simulink subsystem "Vehicle_Model"  (R2022b)
settings: Solver=VariableStepAuto  StartTime=0.0  StopTime=10.0  RelTol=1e-3
undefined symbols (not defined in the file): chassis, dZ, F0z, IMU_accel, IMU_gyro, IMU_mag, phi, powertrain, psi, sim, sus, suspension, theta, trn, veh, VEH, whl, X, Xdot, Y, Ydot, Z, Zdot
libraries: fl_lib x53, nesl_utility x15, vehdynlibtire x10, vehdynlibsuspension x8, EngineCoolingComponents_lib x5, autolibutils x5, sharedtransform x5, shared6dof x2, sensorgpslib x1, mspsensorlib x1, dspstat3 x1, SimscapeFluids_lib x1
(part 8 of 8)

== system Vehicle_Model/Wheels and Tires/VDBS/Tires/MF Tires Vector ==
  DriveTorque : Inport
  Brake Pedal : Inport  Port=2
  r : Inport  Port=3
  Vx : Inport  Port=4
  Vy : Inport  Port=5
  Camber : Inport  Port=6
  Press : Inport  Port=7  Unit=Pa
  lambda : Inport  Port=8  Unit=1
  Gnd : Inport  Port=9
  FzSusp : Inport  Port=10
  Combined Slip Wheel 2DOF : vehdynlibtire/Combined Slip Wheel 2DOF  plySteer=on  turnslip=on  tireType=External file  BrakeType=Disc  mu_static=powertrain.brake.mu_static  mu_kinetic=powertrain.brake.mu_kinetic  disk_abore=powertrain.brake.disk_abore  Rm=powertrain.brake.Rm  num_pads=powertrain.brake.num_pads  drum_abore=0.0508  drum_a=0.123  drum_c=0.212  drum_r=0.15  drum_theta1=0  drum_theta2=126  brake_p_bpt=[1 11.4736842105263 21.9473684210526 32.4210526315789 42.8947368421053 53.3684210526316 63.8421052631579 74.3157894736842 84.7894736842105 95.2631578947368 105.736842105263 116.210526315789 126.684210526316 137.157894736842 147.631578947368 158.105263157895 168.578947368421 179.052631578947 189.526315789474 200]  brake_n_bpt=[0 52.6315789473684 105.263157894737 157.894736842105 210.526315789474 263.157894736842 315.789473684211 368.421052631579 421.052631578947 473.684210526316 526.315789473684 578.947368421053 631.578947368421 684.210526315789 736.842105263158 789.473684210526 842.105263157895 894.736842105263 947.368421052632 1000]  f_brake_t=[43.4900602404453 42.5056030554862 41.5350898940194 40.5780454442085 39.6340111501808 38.7025443887544 37.7832176914519 36.8756180088306 35.9793460143796 35.0940154454303 34.2192524787115 33.3546951383474 32.4999927342521 31.6548053290159 30.8188032315107 29.991666515561 29.1730845621415 28.362755623661 27.5603864089927 26.765691687993;498.991217495636 487.695866636631 476.560505099801 465.579679307235 454.748127933653 444.060772460445 433.51270824929 423.099196101319 412.81565427025 402.657650900201 392.620896861006 382.701238955775 372.894653477208 363.197240090814 353.605216024701 344.114910546964 334.722759712992 325.425301366216 316.219170376863 307.10109410434;954.492374750826 932.886130217776 911.585920305583 890.581313170261 869.862244717126 849.419000532136 829.242198807128 809.322774193808 789.651962526121 770.221286354971 751.0225412433 732.047782773203 713.289314220164 694.739674852612 676.391628817892 658.238154578366 640.272434863842 622.48784710877 604.877954344734 587.436496520688;1409.99353200602 1378.07639379892 1346.61133551136 1315.58294703329 1284.9763615006 1254.77722860383 1224.97168936497 1195.5463522863 1166.48827078199 1137.78492180974 1109.42418562559 1081.39432659063 1053.68397496312 1026.28210961441 999.178041611083 972.361398609768 945.822110014692 919.550392851325 893.536738312604 867.771898937035;1865.49468926121 1823.26665738007 1781.63675071715 1740.58458089631 1700.09047828407 1660.13545667552 1620.7011799228 1581.76993037878 1543.32457903786 1505.34855726451 1467.82583000789 1430.74087040806 1394.07863570608 1357.82454437621 1321.96445440427 1286.48464264117 1251.37178516554 1216.61293859388 1182.19552228048 1148.10730135338;2320.9958465164 2268.45692096121 2216.66216592293 2165.58621475934 2115.20459506754 2065.49368474721 2016.43067048064 1967.99350847127 1920.16088729373 1872.91219271928 1826.22747439018 1780.08741422549 1734.47329644903 1689.36697913801 1644.75086719747 1600.60788667257 1556.92146031639 1513.67548433643 1470.85430624835 1428.44270376973;2776.49700377159 2713.64718454235 2651.68758112871 2590.58784862237 2530.31871185102 2470.8519128189 2412.16016103848 2354.21708656376 2296.9971955496 2240.47582817405 2184.62911877248 2129.43395804292 2074.86795719199 2020.9094138998 1967.53727999066 1914.73113070398 1862.47113546724 1810.73803007899 1759.51309021622 1708.77810618608;3231.99816102678 3158.8374481235 3086.71299633449 3015.58948248539 2945.43282863449 2876.21014089059 2807.88965159632 2740.44066465625 2673.83350380547 2608.03946362882 2543.03076315477 2478.78050186034 2415.26261793494 2352.4518486616 2290.32369278385 2228.85437473538 2168.02081061809 2107.80057582154 2048.17187418409 1989.11350860242;3687.49931828197 3604.02771170464 3521.73841154027 3440.59111634842 3360.54694541796 3281.56836896228 3203.61914215416 3126.66424274874 3050.66981206134 2975.60309908359 2901.43240753707 2828.12704567777 2755.6572786779 2683.9942834234 2613.11010557704 2542.97761876678 2473.57048576894 2404.8631215641 2336.83065815196 2269.44891101877;4143.00047553716 4049.21797528579 3956.76382674606 3865.59275021144 3775.66106220143 3686.92659703397 3599.34863271199 3512.88782084123 3427.50612031721 3343.16673453836 3259.83405191936 3177.4735894952 3096.05193942085 3015.5367181852 2935.89651837023 2857.10086279818 2779.12016091979 2701.92566730665 2625.48944211983 2549.78431343512;4598.50163279235 4494.40823886693 4391.78924195184 4290.59438407447 4190.77517898491 4092.28482510566 3995.07812326983 3899.11139893372 3804.34242857308 3710.73036999313 3618.23569630166 3526.82013331263 3436.44660016381 3347.079152947 3258.68293116342 3171.22410682959 3084.66983607064 2998.98821304921 2914.1482260877 2830.11971585147;5054.00279004754 4939.59850244808 4826.81465715762 4715.59601793749 4605.88929576838 4497.64305317735 4390.80761382767 4285.3349770262 4181.17873682896 4078.2940054479 3976.63734068395 3876.16667713006 3776.84126090677 3678.62158770879 3581.46934395661 3485.34735086099 ...(+2764 chars)]  tireParamSet=C:\Users\Inver\Documents\GitHub\SimscapeModel\Vehicle Parameters\PROCESSED_DATA\Round_6_Hoosier_LCO_18x6_10_on_6in_12psi_PAC02_UM4.tir  PRESMAX=1000000  PRESMIN=10000  FZMAX=1121  FZMIN=10  VXLOW=1  KPUMAX=0.25  KPUMIN=-0.25  ALPMAX=0.261799  ALPMIN=-0.261799  CAMMAX=0.069813  CAMMIN=-0.069813  LONGVL=11.176  FxRelFreqLwrLim=200*pi  FyRelFreqLwrLim=50*pi  MyRelFreqLwrLim=100*pi  omegao=sim.IC.omega_IC  br=suspension.tire.br  UNLOADED_RADIUS=0.2286  NOMPRES=sim.strange_parameters.NOMPRES  FNOMIN=601  WIDTH=0.1524  RIM_RADIUS=0.127  MASS=mean(chassis.mass.m_unsprung)  IYY=suspension.tire.IYY  GRAVITY=-sim.constant.g  zo=sim.IC.z_tire_IC  zdoto=sim.IC.zdot_tires_IC  BREFF=2.49297  DREFF=0.321682  FREFF=0.251668  Q_RE0=1.00866439868088  Q_V1=0.000760413786224011  Q_V2=0.0463384792019201  Q_FZ1=0  Q_FZ2=15.6870832810226  Q_FZ3=0  Q_FCX=0.138643970247602  Q_FCY=0.10843499565426  Q_FCY2=-0.465763352339538  PFZ1=0.69958166705601  VERTICAL_STIFFNESS=112400  VERTICAL_DAMPING=118.254  BOTTOM_OFFST=0.00990653336182505  BOTTOM_STIFF=1999075.87051971  LONGITUDINAL_STIFFNESS=388714.175879854  LATERAL_STIFFNESS=157087.404633332  PCFX1=0.18539229191199  PCFX2=0  PCFX3=0  PCFY1=0.163183345037677  PCFY2=0  PCFY3=0.249094918231954  Q_RA1=0.675942571700787  Q_RA2=0.73800463546164  Q_RB1=1.04487486456705  Q_RB2=-1.191763806629  PCX1=0.966202  PDX1=2.80407  PDX2=-0.357084  PDX3=6.84244  PEX1=-6.80827e-05  PEX2=-1.03475  PEX3=-0.53468  PEX4=-1  PKX1=54.4164  PKX2=-22.3491  PKX3=0.0455377  PHX1=0.00128776  PHX2=0.00137717  PVX1=-0.0646749  PVX2=-0.100465  PPX1=0  PPX2=0  PPX3=0  PPX4=0  RBX1=100  RBX2=44.8344  RBX3=0  RCX1=0.856322  REX1=0.518432  REX2=0.240784  RHX1=-0.0150667  QSX1=-0.0194497  QSX2=-1.24676  QSX3=0.000838911  QSX4=0.807548  QSX5=-0.37375  QSX6=1.16556  QSX7=-5.15598  QSX8=-0.492061  QSX9=-0.177936  QSX10=1  QSX11=0.888738  QSX12=0  QSX13=0  QSX14=0  PPMX1=0  PCY1=0.752535  PDY1=-3.27392  PDY2=0.218557  PDY3=6.02342  PEY1=0  PEY2=0.252909  PEY3=-0.706443  PEY4=0.9  PEY5=0  PKY1=-48.6492  PKY2=1.68896  PKY3=1.62566  PKY4=1.98176755955416  PKY5=0  PKY6=-0.884005199550313  PKY7=-0.237259727611847  PHY1=0.0017727  PHY2=-0.00215785  PVY1=0.0212074  PVY2=-0.0480939  PVY3=0.200755  PVY4=-1.48156  PPY1=0  PPY2=0  PPY3=0  PPY4=0  PPY5=0  RBY1=12.042  RBY2=10.4  RBY3=-0.0251847  RBY4=0  RCY1=1.05268  REY1=-0.0970159  REY2=-0.211702  RHY1=0.00468209  RHY2=0.0130759  RVY1=0.00281892  RVY2=-0.0024726  RVY3=-0.0308756  RVY4=-50  RVY5=-3  RVY6=22  QSY1=0  QSY2=0  QSY3=0  QSY4=0  QSY5=0  QSY6=0  QSY7=0  QSY8=0  QBZ1=7.76297  QBZ2=1.09215  QBZ3=-0.949071  QBZ4=9.45639  QBZ5=-9.95728  QBZ6=0  QBZ9=0  QBZ10=2.46233  QCZ1=1.1619  QDZ1=0.130674  QDZ2=-0.0191515  QDZ3=-2.11221  QDZ4=4.36886  QDZ6=0.00252395  QDZ7=0.0164922  QDZ8=-1.57877  QDZ9=0.435267  QDZ10=0  QDZ11=0  QEZ1=-2.11897  QEZ2=0.850576  QEZ3=0.223032  QEZ4=0.657831  QEZ5=-7.10343  QHZ1=0.00740081  QHZ2=-0.00996544  QHZ3=0.0623105  QHZ4=-0.331019  PPZ1=-0.443927982388615  PPZ2=0  SSZ1=-0.0881802  SSZ2=-0.0389434  SSZ3=1.55783  SSZ4=-0.570516  PDXP1=0.396718274678791  PDXP2=0  PDXP3=0  PKYP1=1.00587060633573  PDYP1=0.40483048923438  PDYP2=0  PDYP3=0  PDYP4=0  PHYP1=0.992731942067188  PHYP2=0.150352945499914  PHYP3=0  PHYP4=-3.98988682633674  PECP1=0.502379254513503  PECP2=0  QDTP1=10.0178654287947  QCRP1=0.200627747200702  QCRP2=0.0995735881599772  QBRP1=0.0997107127960717  QDRP1=1.01432910167423  QDRP2=0  aMode=2
  Terminator{7..13} (7 alike) : Terminator
  Wheels : Outport  VectorParamsAs1DForOutWhenUnconnected=off
  wires:
  lambda/1 -> Combined Slip Wheel 2DOF/10
  Combined Slip Wheel 2DOF/1 -> Wheels/1
  DriveTorque/1 -> Combined Slip Wheel 2DOF/2
  Vx/1 -> Combined Slip Wheel 2DOF/3
  Camber/1 -> Combined Slip Wheel 2DOF/5
  r/1 -> Combined Slip Wheel 2DOF/6
  Press/1 -> Combined Slip Wheel 2DOF/7
  Gnd/1 -> Combined Slip Wheel 2DOF/8
  FzSusp/1 -> Combined Slip Wheel 2DOF/9
  Combined Slip Wheel 2DOF/2 -> Terminator7/1
  Combined Slip Wheel 2DOF/3 -> Terminator8/1
  Combined Slip Wheel 2DOF/4 -> Terminator9/1
  Combined Slip Wheel 2DOF/5 -> Terminator10/1
  Combined Slip Wheel 2DOF/6 -> Terminator11/1
  Combined Slip Wheel 2DOF/7 -> Terminator12/1
  Combined Slip Wheel 2DOF/8 -> Terminator13/1
  Vy/1 -> Combined Slip Wheel 2DOF/4
  Brake Pedal/1 -> Combined Slip Wheel 2DOF/1

== system Vehicle_Model/Wheels and Tires/VDBS/Veh2Tire/Wheel Angles ==
  steer : Inport
  camber : Inport  Port=2
  Constant3 : Constant  Value=ones(1,4).*0
  Reshape : Reshape  OutputDimensionality=Row vector (2-D)
  Reshape1 : Reshape  OutputDimensionality=Row vector (2-D)
  Reshape2 : Reshape  OutputDimensionality=Row vector (2-D)
  Vector Concatenate3 : Concatenate  NumInputs=3  Mode=Multidimensional array
  Vehicle : Outport  VectorParamsAs1DForOutWhenUnconnected=off
  wires:
  Constant3/1 -> Reshape2/1
  Vector Concatenate3/1 -> Vehicle/1
  Reshape/1 -> Vector Concatenate3/3
  Reshape1/1 -> Vector Concatenate3/1
  camber/1 -> Reshape1/1
  Reshape2/1 -> Vector Concatenate3/2
  steer/1 -> Reshape/1

== system Vehicle_Model/Wheels and Tires/VDBS/Veh2Tire/Wheel to Body Transform ==
  VelVeh : Inport  Partition=on  PartitionDimension=2  PartitionWidth=1  PartitionOffset=0
  WheelAngles : Inport  Port=2  Partition=on  PartitionDimension=2  PartitionWidth=1  PartitionOffset=0
  Constant : Constant  Value=[pi;0;0]
  Demux1 : Demux  Outputs=3
  Divide1 : Product  Inputs=**  Multiplication=Matrix(*)
  Divide2 : Product  Inputs=**  Multiplication=Matrix(*)
  For Each : ForEach  DisableCoverage=on
  Rotation Angles to Direction Cosine Matrix : sharedtransform/Rotation Angles to Direction Cosine Matrix  rotationOrder=ZYX  aMode=2
  Rotation Angles to Direction Cosine Matrix1 : sharedtransform/Rotation Angles to Direction Cosine Matrix  rotationOrder=ZYX  aMode=2
  Selector : Selector  InputPortWidth=3  IndexOptions=Index vector (dialog)  Indices=[3 2 1]  OutputSizes=1
  Selector1 : Selector  InputPortWidth=3  IndexOptions=Index vector (dialog)  Indices=[3 2 1]  OutputSizes=1
  xdotWheel : Outport  ConcatenationDimension=1  VectorParamsAs1DForOutWhenUnconnected=off
  ydotWheel : Outport  Port=2  ConcatenationDimension=1  VectorParamsAs1DForOutWhenUnconnected=off
  zdotWheel : Outport  Port=3  ConcatenationDimension=1  VectorParamsAs1DForOutWhenUnconnected=off
  wires:
  Divide2/1 -> Demux1/1
  Demux1/1 -> xdotWheel/1
  Demux1/2 -> ydotWheel/1
  Demux1/3 -> zdotWheel/1
  Rotation Angles to Direction Cosine Matrix/1 -> Divide1/1
  VelVeh/1 -> Divide1/2
  WheelAngles/1 -> Selector/1
  Selector/1 -> Rotation Angles to Direction Cosine Matrix/1
  Selector1/1 -> Rotation Angles to Direction Cosine Matrix1/1
  Rotation Angles to Direction Cosine Matrix1/1 -> Divide2/1
  Divide1/1 -> Divide2/2
  Constant/1 -> Selector1/1

== system Vehicle_Model/Wheels and Tires/VDBS/Tires/Fiala Tires/Fx ==
  In1 : Inport
  In2 : Inport  Port=2
  In3 : Inport  Port=3
  In4 : Inport  Port=4
  Bus Selector{,1..3} (4 alike) : BusSelector  OutputSignals=Fx
  Vector Concatenate : Concatenate  NumInputs=4
  Out1 : Outport  VectorParamsAs1DForOutWhenUnconnected=off
  wires:
  Bus Selector3/1 -> Vector Concatenate/4  "<Fx>"
  Bus Selector2/1 -> Vector Concatenate/3  "<Fx>"
  Bus Selector1/1 -> Vector Concatenate/2  "<Fx>"
  In4/1 -> Bus Selector3/1
  In3/1 -> Bus Selector2/1
  In2/1 -> Bus Selector1/1
  Bus Selector/1 -> Vector Concatenate/1  "<Fx>"
  In1/1 -> Bus Selector/1
  Vector Concatenate/1 -> Out1/1

== system Vehicle_Model/Wheels and Tires/VDBS/Tires/Fiala Tires/Fy ==
  In1 : Inport
  In2 : Inport  Port=2
  In3 : Inport  Port=3
  In4 : Inport  Port=4
  Bus Selector{,1..3} (4 alike) : BusSelector  OutputSignals=Fy
  Vector Concatenate : Concatenate  NumInputs=4
  Out1 : Outport  VectorParamsAs1DForOutWhenUnconnected=off
  wires:
  Vector Concatenate/1 -> Out1/1
  In1/1 -> Bus Selector/1
  Bus Selector/1 -> Vector Concatenate/1  "<Fy>"
  In2/1 -> Bus Selector1/1
  In3/1 -> Bus Selector2/1
  In4/1 -> Bus Selector3/1
  Bus Selector1/1 -> Vector Concatenate/2  "<Fy>"
  Bus Selector2/1 -> Vector Concatenate/3  "<Fy>"
  Bus Selector3/1 -> Vector Concatenate/4  "<Fy>"

== system Vehicle_Model/Wheels and Tires/VDBS/Tires/Fiala Tires/Fz ==
  In1 : Inport
  In2 : Inport  Port=2
  In3 : Inport  Port=3
  In4 : Inport  Port=4
  Bus Selector{,1..3} (4 alike) : BusSelector  OutputSignals=Fz
  Vector Concatenate : Concatenate  NumInputs=4
  Out1 : Outport  VectorParamsAs1DForOutWhenUnconnected=off
  wires:
  Vector Concatenate/1 -> Out1/1
  In1/1 -> Bus Selector/1
  Bus Selector/1 -> Vector Concatenate/1  "<Fz>"
  In2/1 -> Bus Selector1/1
  In3/1 -> Bus Selector2/1
  In4/1 -> Bus Selector3/1
  Bus Selector1/1 -> Vector Concatenate/2  "<Fz>"
  Bus Selector2/1 -> Vector Concatenate/3  "<Fz>"
  Bus Selector3/1 -> Vector Concatenate/4  "<Fz>"

== system Vehicle_Model/Wheels and Tires/VDBS/Tires/Fiala Tires/Mx ==
  In1 : Inport
  In2 : Inport  Port=2
  In3 : Inport  Port=3
  In4 : Inport  Port=4
  Bus Selector{,1..3} (4 alike) : BusSelector  OutputSignals=Mx
  Vector Concatenate : Concatenate  NumInputs=4
  Out1 : Outport  VectorParamsAs1DForOutWhenUnconnected=off
  wires:
  Vector Concatenate/1 -> Out1/1
  In1/1 -> Bus Selector/1
  Bus Selector/1 -> Vector Concatenate/1  "<Mx>"
  In2/1 -> Bus Selector1/1
  In3/1 -> Bus Selector2/1
  In4/1 -> Bus Selector3/1
  Bus Selector1/1 -> Vector Concatenate/2  "<Mx>"
  Bus Selector2/1 -> Vector Concatenate/3  "<Mx>"
  Bus Selector3/1 -> Vector Concatenate/4  "<Mx>"

== system Vehicle_Model/Wheels and Tires/VDBS/Tires/Fiala Tires/My ==
  In1 : Inport
  In2 : Inport  Port=2
  In3 : Inport  Port=3
  In4 : Inport  Port=4
  Bus Selector{,1..3} (4 alike) : BusSelector  OutputSignals=My
  Vector Concatenate : Concatenate  NumInputs=4
  Out1 : Outport  VectorParamsAs1DForOutWhenUnconnected=off
  wires:
  Bus Selector3/1 -> Vector Concatenate/4  "<My>"
  Bus Selector2/1 -> Vector Concatenate/3  "<My>"
  Bus Selector1/1 -> Vector Concatenate/2  "<My>"
  In4/1 -> Bus Selector3/1
  In3/1 -> Bus Selector2/1
  In2/1 -> Bus Selector1/1
  Bus Selector/1 -> Vector Concatenate/1  "<My>"
  In1/1 -> Bus Selector/1
  Vector Concatenate/1 -> Out1/1

== system Vehicle_Model/Wheels and Tires/VDBS/Tires/Fiala Tires/Mz ==
  In1 : Inport
  In2 : Inport  Port=2
  In3 : Inport  Port=3
  In4 : Inport  Port=4
  Bus Selector{,1..3} (4 alike) : BusSelector  OutputSignals=Mz
  Vector Concatenate : Concatenate  NumInputs=4
  Out1 : Outport  VectorParamsAs1DForOutWhenUnconnected=off
  wires:
  Bus Selector3/1 -> Vector Concatenate/4  "<Mz>"
  Bus Selector2/1 -> Vector Concatenate/3  "<Mz>"
  Bus Selector1/1 -> Vector Concatenate/2  "<Mz>"
  In4/1 -> Bus Selector3/1
  In3/1 -> Bus Selector2/1
  In2/1 -> Bus Selector1/1
  Bus Selector/1 -> Vector Concatenate/1  "<Mz>"
  In1/1 -> Bus Selector/1
  Vector Concatenate/1 -> Out1/1

== system Vehicle_Model/Wheels and Tires/VDBS/Tires/Fiala Tires/Re ==
  In1 : Inport
  In2 : Inport  Port=2
  In3 : Inport  Port=3
  In4 : Inport  Port=4
  Bus Selector{,1..3} (4 alike) : BusSelector  OutputSignals=Re
  Vector Concatenate : Concatenate  NumInputs=4
  Out1 : Outport  VectorParamsAs1DForOutWhenUnconnected=off
  wires:
  Vector Concatenate/1 -> Out1/1
  In1/1 -> Bus Selector/1
  Bus Selector/1 -> Vector Concatenate/1  "<Re>"
  In2/1 -> Bus Selector1/1
  In3/1 -> Bus Selector2/1
  In4/1 -> Bus Selector3/1
  Bus Selector1/1 -> Vector Concatenate/2  "<Re>"
  Bus Selector2/1 -> Vector Concatenate/3  "<Re>"
  Bus Selector3/1 -> Vector Concatenate/4  "<Re>"

== system Vehicle_Model/Wheels and Tires/VDBS/Tires/Fiala Tires/alpha ==
  In1 : Inport
  In2 : Inport  Port=2
  In3 : Inport  Port=3
  In4 : Inport  Port=4
  Bus Selector{,1..3} (4 alike) : BusSelector  OutputSignals=Alpha
  Vector Concatenate : Concatenate  NumInputs=4
  Out1 : Outport  VectorParamsAs1DForOutWhenUnconnected=off
  wires:
  Vector Concatenate/1 -> Out1/1
  In1/1 -> Bus Selector/1
  Bus Selector/1 -> Vector Concatenate/1  "<Alpha>"
  In2/1 -> Bus Selector1/1
  In3/1 -> Bus Selector2/1
  In4/1 -> Bus Selector3/1
  Bus Selector1/1 -> Vector Concatenate/2  "<Alpha>"
  Bus Selector2/1 -> Vector Concatenate/3  "<Alpha>"
  Bus Selector3/1 -> Vector Concatenate/4  "<Alpha>"

== system Vehicle_Model/Wheels and Tires/VDBS/Tires/Fiala Tires/kappa ==
  In1 : Inport
  In2 : Inport  Port=2
  In3 : Inport  Port=3
  In4 : Inport  Port=4
  Bus Selector{,1..3} (4 alike) : BusSelector  OutputSignals=Kappa
  Vector Concatenate : Concatenate  NumInputs=4
  Out1 : Outport  VectorParamsAs1DForOutWhenUnconnected=off
  wires:
  Bus Selector3/1 -> Vector Concatenate/4  "<Kappa>"
  Bus Selector2/1 -> Vector Concatenate/3  "<Kappa>"
  Bus Selector1/1 -> Vector Concatenate/2  "<Kappa>"
  In4/1 -> Bus Selector3/1
  In3/1 -> Bus Selector2/1
  In2/1 -> Bus Selector1/1
  Bus Selector/1 -> Vector Concatenate/1  "<Kappa>"
  In1/1 -> Bus Selector/1
  Vector Concatenate/1 -> Out1/1

== system Vehicle_Model/Wheels and Tires/VDBS/Tires/Fiala Tires/omega ==
  In1 : Inport
  In2 : Inport  Port=2
  In3 : Inport  Port=3
  In4 : Inport  Port=4
  Bus Selector{,1..3} (4 alike) : BusSelector  OutputSignals=Omega
  Vector Concatenate : Concatenate  NumInputs=4
  Out1 : Outport  VectorParamsAs1DForOutWhenUnconnected=off
  wires:
  In1/1 -> Bus Selector/1
  Bus Selector/1 -> Vector Concatenate/1  "<Omega>"
  In2/1 -> Bus Selector1/1
  In3/1 -> Bus Selector2/1
  In4/1 -> Bus Selector3/1
  Bus Selector1/1 -> Vector Concatenate/2  "<Omega>"
  Bus Selector2/1 -> Vector Concatenate/3  "<Omega>"
  Bus Selector3/1 -> Vector Concatenate/4  "<Omega>"
  Vector Concatenate/1 -> Out1/1

== system Vehicle_Model/Wheels and Tires/VDBS/Tires/Fiala Tires/z ==
  In1 : Inport
  In2 : Inport  Port=2
  In3 : Inport  Port=3
  In4 : Inport  Port=4
  Bus Selector{,1..3} (4 alike) : BusSelector  OutputSignals=z
  Vector Concatenate : Concatenate  NumInputs=4
  Out1 : Outport  VectorParamsAs1DForOutWhenUnconnected=off
  wires:
  Bus Selector3/1 -> Vector Concatenate/4  "<z>"
  Bus Selector2/1 -> Vector Concatenate/3  "<z>"
  Bus Selector1/1 -> Vector Concatenate/2  "<z>"
  In4/1 -> Bus Selector3/1
  In3/1 -> Bus Selector2/1
  In2/1 -> Bus Selector1/1
  Bus Selector/1 -> Vector Concatenate/1  "<z>"
  In1/1 -> Bus Selector/1
  Vector Concatenate/1 -> Out1/1

== system Vehicle_Model/Wheels and Tires/VDBS/Tires/Fiala Tires/zdot ==
  In1 : Inport
  In2 : Inport  Port=2
  In3 : Inport  Port=3
  In4 : Inport  Port=4
  Bus Selector{,1..3} (4 alike) : BusSelector  OutputSignals=zdot
  Vector Concatenate : Concatenate  NumInputs=4
  Out1 : Outport  VectorParamsAs1DForOutWhenUnconnected=off
  wires:
  Vector Concatenate/1 -> Out1/1
  In1/1 -> Bus Selector/1
  Bus Selector/1 -> Vector Concatenate/1  "<zdot>"
  In2/1 -> Bus Selector1/1
  In3/1 -> Bus Selector2/1
  In4/1 -> Bus Selector3/1
  Bus Selector1/1 -> Vector Concatenate/2  "<zdot>"
  Bus Selector2/1 -> Vector Concatenate/3  "<zdot>"
  Bus Selector3/1 -> Vector Concatenate/4  "<zdot>"

== system Vehicle_Model/Wheels and Tires/VDBS/Tires/MF Tires/Fx ==
  In1 : Inport
  In2 : Inport  Port=2
  In3 : Inport  Port=3
  In4 : Inport  Port=4
  Bus Selector{,1..3} (4 alike) : BusSelector  OutputSignals=Fx
  Vector Concatenate : Concatenate  NumInputs=4
  Out1 : Outport  VectorParamsAs1DForOutWhenUnconnected=off
  wires:
  Bus Selector3/1 -> Vector Concatenate/4  "<Fx>"
  Bus Selector2/1 -> Vector Concatenate/3  "<Fx>"
  Bus Selector1/1 -> Vector Concatenate/2  "<Fx>"
  In4/1 -> Bus Selector3/1
  In3/1 -> Bus Selector2/1
  In2/1 -> Bus Selector1/1
  Bus Selector/1 -> Vector Concatenate/1  "<Fx>"
  In1/1 -> Bus Selector/1
  Vector Concatenate/1 -> Out1/1

== system Vehicle_Model/Wheels and Tires/VDBS/Tires/MF Tires/Fy ==
  In1 : Inport
  In2 : Inport  Port=2
  In3 : Inport  Port=3
  In4 : Inport  Port=4
  Bus Selector{,1..3} (4 alike) : BusSelector  OutputSignals=Fy
  Vector Concatenate : Concatenate  NumInputs=4
  Out1 : Outport  VectorParamsAs1DForOutWhenUnconnected=off
  wires:
  Vector Concatenate/1 -> Out1/1
  In1/1 -> Bus Selector/1
  Bus Selector/1 -> Vector Concatenate/1  "<Fy>"
  In2/1 -> Bus Selector1/1
  In3/1 -> Bus Selector2/1
  In4/1 -> Bus Selector3/1
  Bus Selector1/1 -> Vector Concatenate/2  "<Fy>"
  Bus Selector2/1 -> Vector Concatenate/3  "<Fy>"
  Bus Selector3/1 -> Vector Concatenate/4  "<Fy>"

== system Vehicle_Model/Wheels and Tires/VDBS/Tires/MF Tires/Fz ==
  In1 : Inport
  In2 : Inport  Port=2
  In3 : Inport  Port=3
  In4 : Inport  Port=4
  Bus Selector{,1..3} (4 alike) : BusSelector  OutputSignals=Fz
  Vector Concatenate : Concatenate  NumInputs=4
  Out1 : Outport  VectorParamsAs1DForOutWhenUnconnected=off
  wires:
  Vector Concatenate/1 -> Out1/1
  In1/1 -> Bus Selector/1
  Bus Selector/1 -> Vector Concatenate/1  "<Fz>"
  In2/1 -> Bus Selector1/1
  In3/1 -> Bus Selector2/1
  In4/1 -> Bus Selector3/1
  Bus Selector1/1 -> Vector Concatenate/2  "<Fz>"
  Bus Selector2/1 -> Vector Concatenate/3  "<Fz>"
  Bus Selector3/1 -> Vector Concatenate/4  "<Fz>"

== system Vehicle_Model/Wheels and Tires/VDBS/Tires/MF Tires/Mx ==
  In1 : Inport
  In2 : Inport  Port=2
  In3 : Inport  Port=3
  In4 : Inport  Port=4
  Bus Selector{,1..3} (4 alike) : BusSelector  OutputSignals=Mx
  Vector Concatenate : Concatenate  NumInputs=4
  Out1 : Outport  VectorParamsAs1DForOutWhenUnconnected=off
  wires:
  Vector Concatenate/1 -> Out1/1
  In1/1 -> Bus Selector/1
  Bus Selector/1 -> Vector Concatenate/1  "<Mx>"
  In2/1 -> Bus Selector1/1
  In3/1 -> Bus Selector2/1
  In4/1 -> Bus Selector3/1
  Bus Selector1/1 -> Vector Concatenate/2  "<Mx>"
  Bus Selector2/1 -> Vector Concatenate/3  "<Mx>"
  Bus Selector3/1 -> Vector Concatenate/4  "<Mx>"

== system Vehicle_Model/Wheels and Tires/VDBS/Tires/MF Tires/My ==
  In1 : Inport
  In2 : Inport  Port=2
  In3 : Inport  Port=3
  In4 : Inport  Port=4
  Bus Selector{,1..3} (4 alike) : BusSelector  OutputSignals=My
  Vector Concatenate : Concatenate  NumInputs=4
  Out1 : Outport  VectorParamsAs1DForOutWhenUnconnected=off
  wires:
  Bus Selector3/1 -> Vector Concatenate/4  "<My>"
  Bus Selector2/1 -> Vector Concatenate/3  "<My>"
  Bus Selector1/1 -> Vector Concatenate/2  "<My>"
  In4/1 -> Bus Selector3/1
  In3/1 -> Bus Selector2/1
  In2/1 -> Bus Selector1/1
  Bus Selector/1 -> Vector Concatenate/1  "<My>"
  In1/1 -> Bus Selector/1
  Vector Concatenate/1 -> Out1/1

== system Vehicle_Model/Wheels and Tires/VDBS/Tires/MF Tires/Mz ==
  In1 : Inport
  In2 : Inport  Port=2
  In3 : Inport  Port=3
  In4 : Inport  Port=4
  Bus Selector{,1..3} (4 alike) : BusSelector  OutputSignals=Mz
  Vector Concatenate : Concatenate  NumInputs=4
  Out1 : Outport  VectorParamsAs1DForOutWhenUnconnected=off
  wires:
  Bus Selector3/1 -> Vector Concatenate/4  "<Mz>"
  Bus Selector2/1 -> Vector Concatenate/3  "<Mz>"
  Bus Selector1/1 -> Vector Concatenate/2  "<Mz>"
  In4/1 -> Bus Selector3/1
  In3/1 -> Bus Selector2/1
  In2/1 -> Bus Selector1/1
  Bus Selector/1 -> Vector Concatenate/1  "<Mz>"
  In1/1 -> Bus Selector/1
  Vector Concatenate/1 -> Out1/1

== system Vehicle_Model/Wheels and Tires/VDBS/Tires/MF Tires/Re ==
  In1 : Inport
  In2 : Inport  Port=2
  In3 : Inport  Port=3
  In4 : Inport  Port=4
  Bus Selector{,1..3} (4 alike) : BusSelector  OutputSignals=Re
  Vector Concatenate : Concatenate  NumInputs=4
  Out1 : Outport  VectorParamsAs1DForOutWhenUnconnected=off
  wires:
  Vector Concatenate/1 -> Out1/1
  In1/1 -> Bus Selector/1
  Bus Selector/1 -> Vector Concatenate/1  "<Re>"
  In2/1 -> Bus Selector1/1
  In3/1 -> Bus Selector2/1
  In4/1 -> Bus Selector3/1
  Bus Selector1/1 -> Vector Concatenate/2  "<Re>"
  Bus Selector2/1 -> Vector Concatenate/3  "<Re>"
  Bus Selector3/1 -> Vector Concatenate/4  "<Re>"

== system Vehicle_Model/Wheels and Tires/VDBS/Tires/MF Tires/alpha ==
  In1 : Inport
  In2 : Inport  Port=2
  In3 : Inport  Port=3
  In4 : Inport  Port=4
  Bus Selector{,1..3} (4 alike) : BusSelector  OutputSignals=Alpha
  Vector Concatenate : Concatenate  NumInputs=4
  Out1 : Outport  VectorParamsAs1DForOutWhenUnconnected=off
  wires:
  Vector Concatenate/1 -> Out1/1
  In1/1 -> Bus Selector/1
  Bus Selector/1 -> Vector Concatenate/1  "<Alpha>"
  In2/1 -> Bus Selector1/1
  In3/1 -> Bus Selector2/1
  In4/1 -> Bus Selector3/1
  Bus Selector1/1 -> Vector Concatenate/2  "<Alpha>"
  Bus Selector2/1 -> Vector Concatenate/3  "<Alpha>"
  Bus Selector3/1 -> Vector Concatenate/4  "<Alpha>"

== system Vehicle_Model/Wheels and Tires/VDBS/Tires/MF Tires/kappa ==
  In1 : Inport
  In2 : Inport  Port=2
  In3 : Inport  Port=3
  In4 : Inport  Port=4
  Bus Selector{,1..3} (4 alike) : BusSelector  OutputSignals=Kappa
  Vector Concatenate : Concatenate  NumInputs=4
  Out1 : Outport  VectorParamsAs1DForOutWhenUnconnected=off
  wires:
  Bus Selector3/1 -> Vector Concatenate/4  "<Kappa>"
  Bus Selector2/1 -> Vector Concatenate/3  "<Kappa>"
  Bus Selector1/1 -> Vector Concatenate/2  "<Kappa>"
  In4/1 -> Bus Selector3/1
  In3/1 -> Bus Selector2/1
  In2/1 -> Bus Selector1/1
  Bus Selector/1 -> Vector Concatenate/1  "<Kappa>"
  In1/1 -> Bus Selector/1
  Vector Concatenate/1 -> Out1/1

== system Vehicle_Model/Wheels and Tires/VDBS/Tires/MF Tires/omega ==
  In1 : Inport
  In2 : Inport  Port=2
  In3 : Inport  Port=3
  In4 : Inport  Port=4
  Bus Selector{,1..3} (4 alike) : BusSelector  OutputSignals=Omega
  Vector Concatenate : Concatenate  NumInputs=4
  Out1 : Outport  VectorParamsAs1DForOutWhenUnconnected=off
  wires:
  In1/1 -> Bus Selector/1
  Bus Selector/1 -> Vector Concatenate/1  "<Omega>"
  In2/1 -> Bus Selector1/1
  In3/1 -> Bus Selector2/1
  In4/1 -> Bus Selector3/1
  Bus Selector1/1 -> Vector Concatenate/2  "<Omega>"
  Bus Selector2/1 -> Vector Concatenate/3  "<Omega>"
  Bus Selector3/1 -> Vector Concatenate/4  "<Omega>"
  Vector Concatenate/1 -> Out1/1

== system Vehicle_Model/Wheels and Tires/VDBS/Tires/MF Tires/z ==
  In1 : Inport
  In2 : Inport  Port=2
  In3 : Inport  Port=3
  In4 : Inport  Port=4
  Bus Selector{,1..3} (4 alike) : BusSelector  OutputSignals=z
  Vector Concatenate : Concatenate  NumInputs=4
  Out1 : Outport  VectorParamsAs1DForOutWhenUnconnected=off
  wires:
  Bus Selector3/1 -> Vector Concatenate/4  "<z>"
  Bus Selector2/1 -> Vector Concatenate/3  "<z>"
  Bus Selector1/1 -> Vector Concatenate/2  "<z>"
  In4/1 -> Bus Selector3/1
  In3/1 -> Bus Selector2/1
  In2/1 -> Bus Selector1/1
  Bus Selector/1 -> Vector Concatenate/1  "<z>"
  In1/1 -> Bus Selector/1
  Vector Concatenate/1 -> Out1/1

== system Vehicle_Model/Wheels and Tires/VDBS/Tires/MF Tires/zdot ==
  In1 : Inport
  In2 : Inport  Port=2
  In3 : Inport  Port=3
  In4 : Inport  Port=4
  Bus Selector{,1..3} (4 alike) : BusSelector  OutputSignals=zdot
  Vector Concatenate : Concatenate  NumInputs=4
  Out1 : Outport  VectorParamsAs1DForOutWhenUnconnected=off
  wires:
  Vector Concatenate/1 -> Out1/1
  In1/1 -> Bus Selector/1
  Bus Selector/1 -> Vector Concatenate/1  "<zdot>"
  In2/1 -> Bus Selector1/1
  In3/1 -> Bus Selector2/1
  In4/1 -> Bus Selector3/1
  Bus Selector1/1 -> Vector Concatenate/2  "<zdot>"
  Bus Selector2/1 -> Vector Concatenate/3  "<zdot>"
  Bus Selector3/1 -> Vector Concatenate/4  "<zdot>"

== matlab function Vehicle_Model/Vehicle/6DOF/Suspension to Chasiss Transforms/Estimated Unsprung Mass Orientation ==
  data: angles output size=3; angleIn input size=3; GeomXYZ output size=3; GemoXYZIn input size=3; Ground input size=4; trackW parameter; wheelB parameter
function [angles,GeomXYZ]= three26(angleIn, GemoXYZIn, Ground,trackW, wheelB)%#codegen
coder.allowpcode('plain')
% Copyright 2018 The MathWorks, Inc.
[angles,GeomXYZ]= vdynthree2six(angleIn, GemoXYZIn, Ground,trackW, wheelB);

== matlab function Vehicle_Model/Vehicle/6DOF/Suspension to Chasiss Transforms/Downforce ==
  data: u input; y output; sim parameter; chassis parameter
function y = fcn(u, sim, chassis)

Fz = 0.5*sim.constant.rho*chassis.aero.Af*chassis.aero.Cl*u^2;

y = [0 0 Fz];

== matlab function Vehicle_Model/Electronics/Navigation Sensors/VNED to SNED ==
  data: accel_SNED output; gyro_SNED output; accel_VNED input size=[3 1]; gyro_VNED input size=[3 1]; mag_VNED input size=[3 1]; mag_SNED output; chassis parameter
function [accel_SNED, gyro_SNED, mag_SNED] = VNED2SNED(accel_VNED, gyro_VNED, mag_VNED, chassis)
%% Define Rotation
IMUNED2VNED = rotmat(quaternion([0 (chassis.geometry.phi - 180) 0],"eulerd","XYZ","frame"),"frame");
MAGNED2VNED = rotmat(quaternion([180 (180 - chassis.geometry.phi) 0],"eulerd","XYZ","frame"),"frame");

%% Coordinate Transformation
accel_SNED = IMUNED2VNED\accel_VNED;
gyro_SNED = IMUNED2VNED\gyro_VNED;
mag_SNED = MAGNED2VNED\mag_VNED;

end

== matlab function Vehicle_Model/Electronics/Navigation Sensors/integrate angvel ==
  data: Orientation_e input; Orientation_c output; Orientation_e output
function [Orientation_c, Orientation_e]  = fcn(Orientation_e)

Orientation_q = quaternion(Orientation_e', 'euler', 'XYZ', 'frame');

Orientation_c = compact(Orientation_q);

end
